simulink library "DivisionVectorScalar"  (R2014b)
settings: Solver=ode45  StartTime=0.0  StopTime=10.0  RelTol=1e-3
settings Model: Creator=Hp  LastModifiedBy=Hp

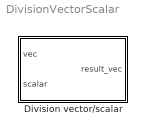
== system DivisionVectorScalar ==
  Division vector/scalar : Subsystem

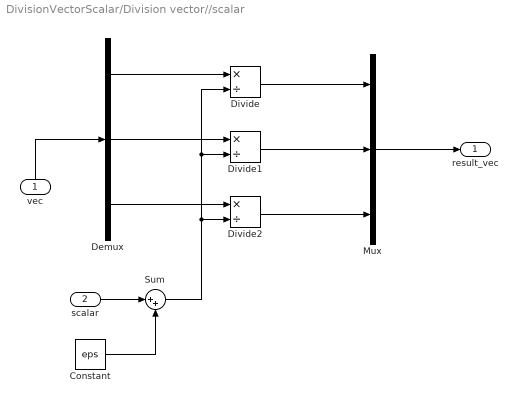
== system DivisionVectorScalar/Division vector//scalar ==
  vec : Inport
  scalar : Inport  Port=2
  Constant : Constant  Value=eps
  Demux : Demux  Outputs=3
  Divide : Product  Inputs=*/
  Divide1 : Product  Inputs=*/
  Divide2 : Product  Inputs=*/
  Mux : Mux  Inputs=3
  Sum : Sum  Inputs=|++
  result_vec : Outport
  wires:
  vec/1 -> Demux/1
  Demux/2 -> Divide1/1
  Demux/1 -> Divide/1
  Divide1/1 -> Mux/2
  Divide2/1 -> Mux/3
  Demux/3 -> Divide2/1
  Sum/1 -> Divide2/2, Divide/2, Divide1/2
  Mux/1 -> result_vec/1
  Divide/1 -> Mux/1
  Constant/1 -> Sum/2
  scalar/1 -> Sum/1
